simulink model "AMdemod_bis"  (R2021a)
settings: Solver=VariableStepAuto  StartTime=0.0  StopTime=10.0  RelTol=1e-3
libraries: hdlsllib x5, dspsrcs4 x3
settings Model: Creator=guido  LastModifiedBy=guido
settings OptimizationCC: BlockReduction=off  ConditionallyExecuteInputs=off  DefaultParameterBehavior=Inlined
settings DebuggingCC: AlgebraicLoopMsg=error
settings HardwareCC: ProdBitPerPointer=32  ProdBitPerSizeT=32  ProdBitPerPtrDiffT=32  ProdLargestAtomicFloat=None  ProdIntDivRoundTo=Undefined  ProdEndianess=Unspecified  ProdWordSize=32  ProdHWDeviceType=ASIC/FPGA->ASIC/FPGA  TargetBitPerPointer=64  TargetBitPerSizeT=64  TargetBitPerPtrDiffT=64  TargetLongLongMode=on  TargetIntDivRoundTo=Zero  TargetEndianess=LittleEndian  TargetWordSize=64  TargetHWDeviceType=Custom Processor->MATLAB Host Computer  ProdEqTarget=off

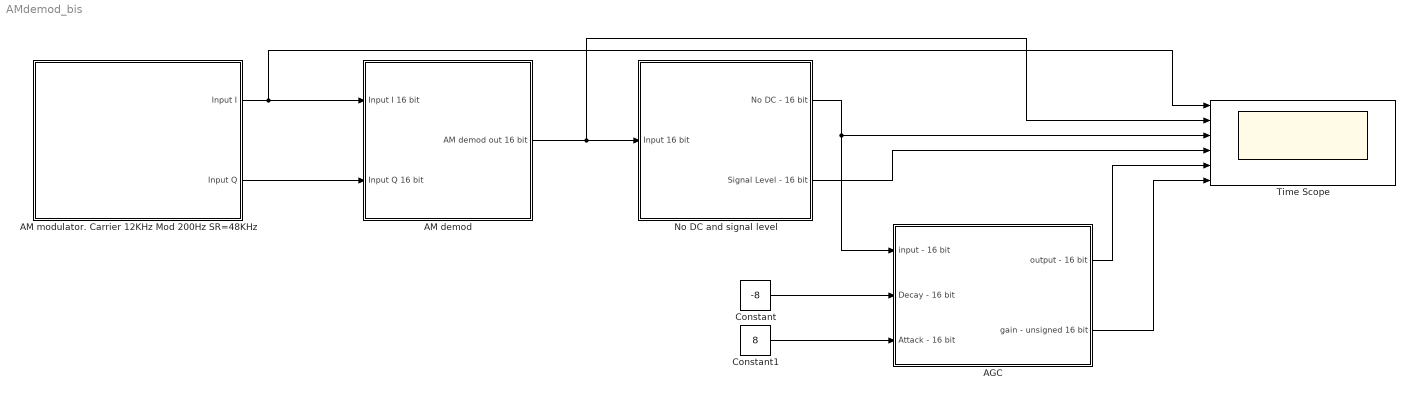
== system AMdemod_bis ==
  AGC : Subsystem
  AM demod : Subsystem
  "AM modulator. Carrier 12KHz Mod 200Hz SR=48KHz " : Subsystem
  Constant : Constant  Value=-8  OutDataTypeStr=int16
  Constant1 : Constant  Value=8  OutDataTypeStr=int16
  No DC and signal level : Subsystem
  Time Scope : Scope  NumInputPorts=6
  wires:
  "AM modulator. Carrier 12KHz Mod 200Hz SR=48KHz "/1(Input I) -> AM demod/1(Input I 16 bit), Time Scope/1
  "AM modulator. Carrier 12KHz Mod 200Hz SR=48KHz "/2(Input Q) -> AM demod/2(Input Q 16 bit)
  AM demod/1(AM demod out 16 bit) -> No DC and signal level/1(Input 16 bit), Time Scope/2
  No DC and signal level/1(No DC - 16 bit) -> AGC/1(input - 16 bit), Time Scope/3
  No DC and signal level/2("Signal Level - 16 bit ") -> Time Scope/4
  Constant1/1 -> AGC/3(Attack - 16 bit)
  Constant/1 -> AGC/2(Decay - 16 bit)
  AGC/1(output - 16 bit) -> Time Scope/5
  AGC/2(gain - unsigned 16 bit) -> Time Scope/6

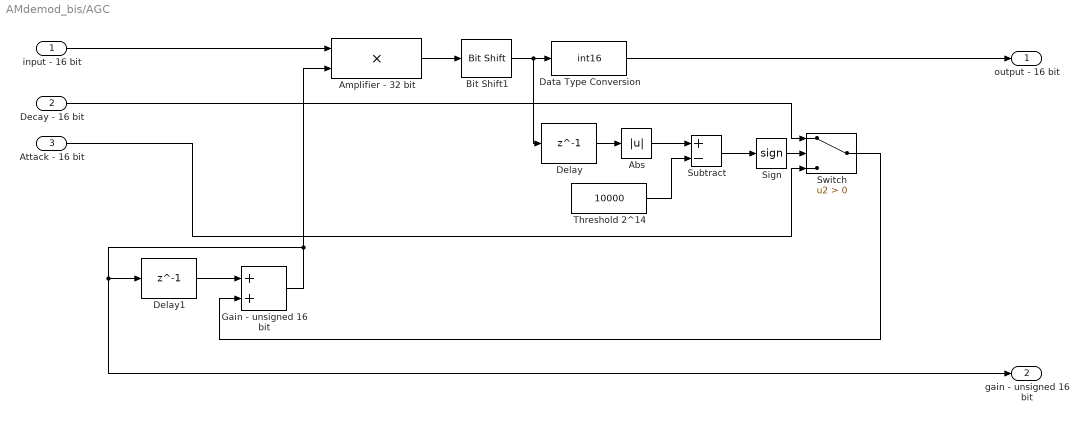
== system AMdemod_bis/AGC ==
  input - 16 bit : Inport  OutDataTypeStr=int16
  Decay - 16 bit : Inport  Port=2  OutDataTypeStr=int16
  Attack - 16 bit : Inport  Port=3  OutDataTypeStr=int16
  Abs : Abs  OutDataTypeStr=int32  SaturateOnIntegerOverflow=on
  Amplifier - 32 bit : Product  OutDataTypeStr=int32  SaturateOnIntegerOverflow=on
  Bit Shift1 : hdlsllib/Logic and Bit Operations/Bit Shift  mode=Shift Right Arithmetic  N=8
  Data Type Conversion : DataTypeConversion  OutDataTypeStr=int16  SaturateOnIntegerOverflow=on
  Delay : Delay  DelayLength=1  InitialCondition=0  UseCircularBuffer=on
  Delay1 : Delay  DelayLength=1  InitialCondition=1  UseCircularBuffer=on
  Gain - unsigned 16 bit : Sum  OutDataTypeStr=fixdt(0,16,0)  SaturateOnIntegerOverflow=on
  Sign : Signum
  Subtract : Sum  Inputs=+-  AccumDataTypeStr=int32  OutDataTypeStr=int32  SaturateOnIntegerOverflow=on
  Switch : Switch  Criteria=u2 > Threshold  OutDataTypeStr=int16  SaturateOnIntegerOverflow=on
  Threshold 2^14 : Constant  Value=10000  OutDataTypeStr=int32
  output - 16 bit : Outport  OutDataTypeStr=int16
  gain - unsigned 16 bit : Outport  Port=2
  wires:
  input - 16 bit/1 -> Amplifier - 32 bit/1
  Delay1/1 -> Gain - unsigned 16 bit/1
  Threshold 2^14/1 -> Subtract/2
  Decay - 16 bit/1 -> Switch/1
  Amplifier - 32 bit/1 -> Bit Shift1/1
  Subtract/1 -> Sign/1
  Attack - 16 bit/1 -> Switch/3
  Sign/1 -> Switch/2
  Abs/1 -> Subtract/1
  Switch/1 -> Gain - unsigned 16 bit/2
  Gain - unsigned 16 bit/1 -> gain - unsigned 16 bit/1, Delay1/1, Amplifier - 32 bit/2
  Delay/1 -> Abs/1
  Data Type Conversion/1 -> output - 16 bit/1
  Bit Shift1/1 -> Delay/1, Data Type Conversion/1

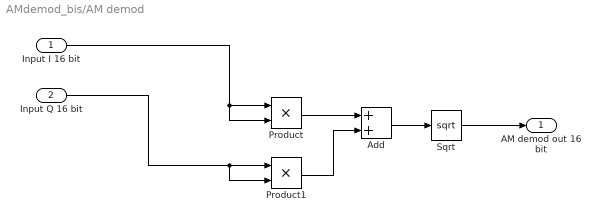
== system AMdemod_bis/AM demod ==
  Input I 16 bit : Inport  OutDataTypeStr=int16
  Input Q 16 bit : Inport  Port=2  OutDataTypeStr=int16
  Add : Sum  OutDataTypeStr=uint32
  Product : Product  OutDataTypeStr=uint32
  Product1 : Product  OutDataTypeStr=uint32
  Sqrt : Sqrt  OutDataTypeStr=int16  SaturateOnIntegerOverflow=on
  AM demod out 16 bit : Outport  OutDataTypeStr=int16
  wires:
  Input Q 16 bit/1 -> Product1/2, Product1/1
  Input I 16 bit/1 -> Product/1, Product/2
  Product1/1 -> Add/2
  Sqrt/1 -> AM demod out 16 bit/1
  Product/1 -> Add/1
  Add/1 -> Sqrt/1

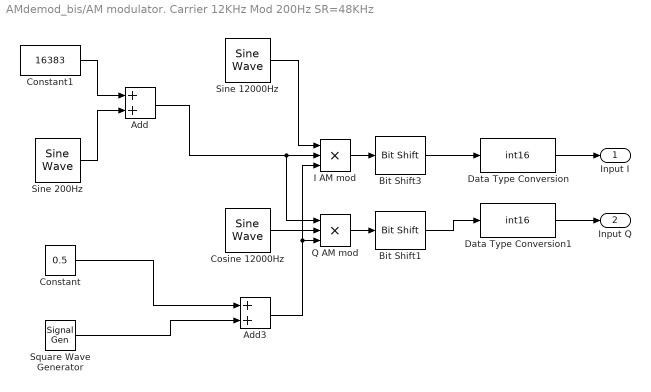
== system AMdemod_bis/AM modulator. Carrier 12KHz Mod 200Hz SR=48KHz  ==
  Add : Sum  AccumDataTypeStr=int16  OutDataTypeStr=int16
  Add3 : Sum
  Bit Shift1 : hdlsllib/Logic and Bit Operations/Bit Shift  mode=Shift Right Arithmetic  N=16
  Bit Shift3 : hdlsllib/Logic and Bit Operations/Bit Shift  mode=Shift Right Arithmetic  N=16
  Constant : Constant  Value=0.5
  Constant1 : Constant  Value=16383  OutDataTypeStr=int16
  Cosine 12000Hz : dspsrcs4/Sine Wave  Amplitude=32767  Frequency=12000  Phase=pi/2  SampleMode=Discrete  OutComplex=Real  CompMethod=Table lookup  TableSize=Speed  SampleTime=1/48000  SamplesPerFrame=1  ResetState=Restart at time zero  OutputFrames=off  dataType=Fixed-point  wordLen=16  udDataType=sfix(16)  fracBitsMode=Best precision  numFracBits=0  OutDataTypeStr=fixdt(1,16)  LastOutDataTypeStr=fixdt(1,16)
  Data Type Conversion : DataTypeConversion  OutDataTypeStr=int16
  Data Type Conversion1 : DataTypeConversion  OutDataTypeStr=int16
  I AM mod : Product  Inputs=3  OutDataTypeStr=int32  SaturateOnIntegerOverflow=on
  Q AM mod : Product  Inputs=3  OutDataTypeStr=int32  SaturateOnIntegerOverflow=on
  Sine 12000Hz : dspsrcs4/Sine Wave  Amplitude=32767  Frequency=12000  Phase=0  SampleMode=Discrete  OutComplex=Real  CompMethod=Table lookup  TableSize=Speed  SampleTime=1/48000  SamplesPerFrame=1  ResetState=Restart at time zero  OutputFrames=off  dataType=Fixed-point  wordLen=16  udDataType=sfix(16)  fracBitsMode=Best precision  numFracBits=0  OutDataTypeStr=fixdt(1,16)  LastOutDataTypeStr=fixdt(1,16)
  Sine 200Hz : dspsrcs4/Sine Wave  Amplitude=16000  Frequency=800  Phase=0  SampleMode=Discrete  OutComplex=Real  CompMethod=Table lookup  TableSize=Speed  SampleTime=1/48000  SamplesPerFrame=1  ResetState=Restart at time zero  OutputFrames=off  dataType=Fixed-point  wordLen=16  udDataType=sfix(16)  fracBitsMode=Best precision  numFracBits=0  OutDataTypeStr=fixdt(1,16)  LastOutDataTypeStr=fixdt(1,16)
  Square Wave Generator : SignalGenerator  WaveForm=square  Amplitude=0.49
  Input I : Outport  OutDataTypeStr=int16
  Input Q : Outport  Port=2  OutDataTypeStr=int16
  wires:
  Q AM mod/1 -> Bit Shift1/1
  I AM mod/1 -> Bit Shift3/1
  Constant1/1 -> Add/1
  Square Wave Generator/1 -> Add3/2
  Sine 200Hz/1 -> Add/2
  Constant/1 -> Add3/1
  Cosine 12000Hz/1 -> Q AM mod/2
  Add/1 -> I AM mod/2, Q AM mod/1
  Sine 12000Hz/1 -> I AM mod/1
  Add3/1 -> Q AM mod/3, I AM mod/3
  Bit Shift3/1 -> Data Type Conversion/1
  Data Type Conversion/1 -> Input I/1
  Bit Shift1/1 -> Data Type Conversion1/1
  Data Type Conversion1/1 -> Input Q/1

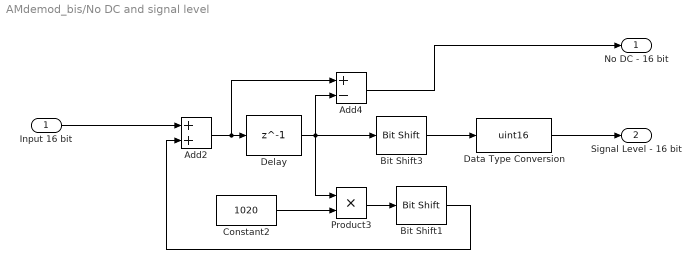
== system AMdemod_bis/No DC and signal level ==
  Input 16 bit : Inport  OutDataTypeStr=int16
  Add2 : Sum  AccumDataTypeStr=int64  OutDataTypeStr=int64
  Add4 : Sum  Inputs=+-  AccumDataTypeStr=int32  OutDataTypeStr=int16
  Bit Shift1 : hdlsllib/Logic and Bit Operations/Bit Shift  mode=Shift Right Arithmetic  N=10
  Bit Shift3 : hdlsllib/Logic and Bit Operations/Bit Shift  mode=Shift Right Arithmetic  N=9
  Constant2 : Constant  Value=1020  OutDataTypeStr=int32
  Data Type Conversion : DataTypeConversion  OutDataTypeStr=uint16
  Delay : Delay  DelayLength=1  InitialCondition=1  UseCircularBuffer=on
  Product3 : Product  OutDataTypeStr=int64
  No DC - 16 bit : Outport
  "Signal Level - 16 bit " : Outport  Port=2  OutDataTypeStr=uint16
  wires:
  Add4/1 -> No DC - 16 bit/1
  Product3/1 -> Bit Shift1/1
  Bit Shift3/1 -> Data Type Conversion/1
  Bit Shift1/1 -> Add2/2
  Add2/1 -> Delay/1, Add4/1
  Input 16 bit/1 -> Add2/1
  Constant2/1 -> Product3/2
  Delay/1 -> Add4/2, Bit Shift3/1, Product3/1
  Data Type Conversion/1 -> "Signal Level - 16 bit "/1
